simulink model "Simulator_Case_7"  (R2024a)
settings: Solver=VariableStepAuto  StartTime=0.0  StopTime=1000  RelTol=1e-3
values from neighbouring files (symbols this model uses):
  Declination_Sigean = 2.116*(pi/180)    (= 0.0369311669722)    [Parametrization_Simulation_Case_7.m]
  Position_Initial_X = Waypoints_X(1)    [Parametrization_Simulation_Case_7.m]
  Position_Initial_Y = Waypoints_Y(1)    [Parametrization_Simulation_Case_7.m]
  Time_Guidance_Sampling = 20    [Parametrization_Simulation_Case_7.m]
  Time_Period_Sampling = 0.1    [Parametrization_Simulation_Case_7.m]
undefined symbols (not defined in the file or in its folder): Area_Lateral_Projected_Wind, Damping_Factor_Waves, Density_Air, Gain_Derivative, Gain_Filter, Gain_Proportional, Inertia_Moment, Length_Ship, Pulsation_Wave, Rudder_Angle_Maximal, Rudder_Angle_Minimal, Rudder_Rate_Maximal, Rudder_Rate_Minimal, Static_Gain_Nomoto, Structure_Wind_Coefficient, Time_Constant_Total, Velocity_Ship_Mean, Wave_Transfer_Function_Discrete, Waypoints, Yaw_Control_Hydrodynamics_Derivative
libraries: simulink_extras x6, cstblocks x2, sensorgpslib x1, sensorinslib x1
(part 1 of 2)
settings Model: Creator=gerar  LastModifiedBy=gerar

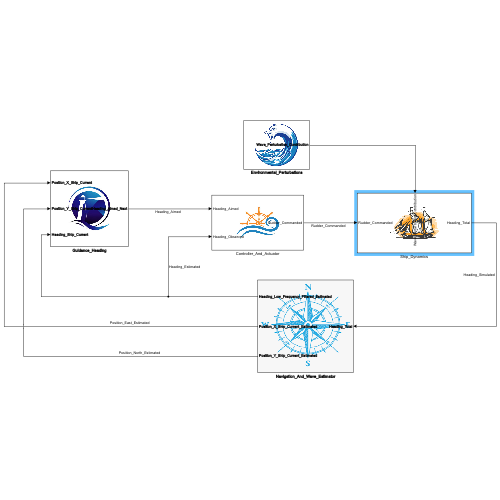
[thumbnail: Simulink's stored preview of the top-level diagram]
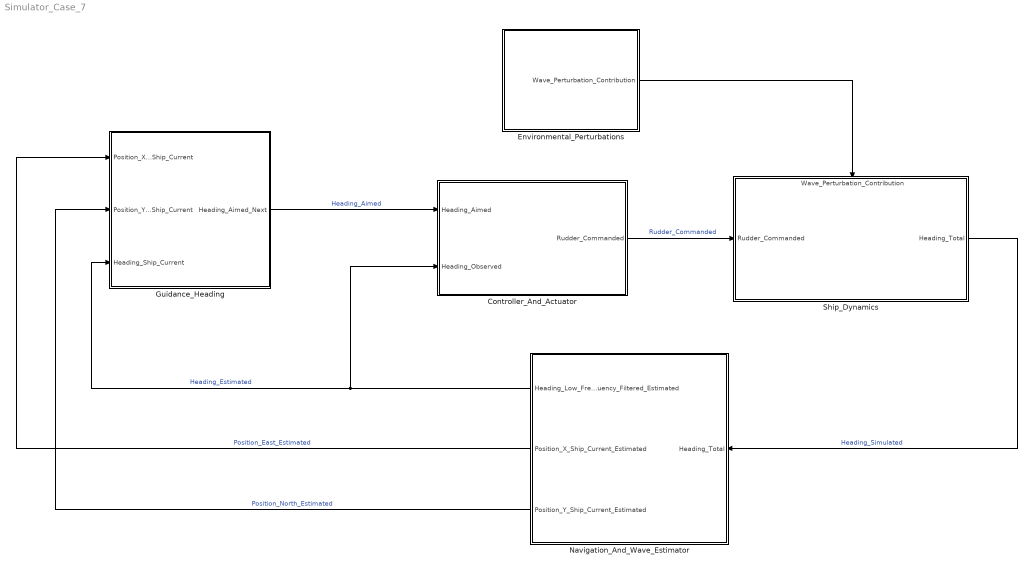
== system Simulator_Case_7 ==
  Controller_And_Actuator : Subsystem
      mask Display: image('Rudder3.jpg');
  Environmental_Perturbations : Subsystem
      mask Display: image('Wave2.png');
  Guidance_Heading : Subsystem
      mask Display: image('phare4.jpg');
  Navigation_And_Wave_Estimator : Subsystem
      mask Display: image('compass4.png');
  Ship_Dynamics : Subsystem
      settings: PortSchema="{\"entries\":[{\"content\":{\"sides\":[{\"content\":{\"connectorIds\":[\"In1\"]},\"type\":\"ConnectorPlacement.EquallySpacedRectSide\",\"uuid\":\"1262d93f-9737-49c5-b1c8-13d3f825160d\"},{\"content\":{\"connectorIds\":[\"Out1\"],\"side\":\"RIGHT\"},\"type\":\"ConnectorPlacement.EquallySpacedRectSide\",\"uuid\":\"2783823e-17f0-4da0-9b4a-e84aa912eb5f\"},{\"content\":{\"connectorIds\":[\"In2\"],\"side\":\"TOP\"},\"type\":\"ConnectorPlacement.EquallySpacedRectSide\",\"uuid\":\"9227960a-c500-4bd1-9392-f2e1de824969\"}]},\"type\":\"ConnectorPlacement.EquallySpacedConnector\",\"uuid\":\"fe1a7a14-057d-49da-982c-994c0d128614\"}],\"packageUris\":[\"http://schema.mathworks.com/mf0/Connector/R2020b\"],\"version\":\"1.0\"}"
      mask Display: image('ship2.png');
  wires:
  Guidance_Heading/1(Heading_Aimed_Next) -> Controller_And_Actuator/1(Heading_Aimed)  "Heading_Aimed"
  Navigation_And_Wave_Estimator/1(Heading_Low_Frequency_Filtered_Estimated) -> Controller_And_Actuator/2(Heading_Observed), Guidance_Heading/3(Heading_Ship_Current)  "Heading_Estimated"
  Environmental_Perturbations/1(Wave_Perturbation_Contribution) -> Ship_Dynamics/2(Wave_Perturbation_Contribution)
  Ship_Dynamics/1(Heading_Total) -> Navigation_And_Wave_Estimator/1(Heading_Total)  "Heading_Simulated"
  Navigation_And_Wave_Estimator/3(Position_Y_Ship_Current_Estimated) -> Guidance_Heading/2(Position_Y_Ship_Current)  "Position_North_Estimated"
  Navigation_And_Wave_Estimator/2(Position_X_Ship_Current_Estimated) -> Guidance_Heading/1(Position_X_Ship_Current)  "Position_East_Estimated"
  Controller_And_Actuator/1(Rudder_Commanded) -> Ship_Dynamics/1(Rudder_Commanded)  "Rudder_Commanded"

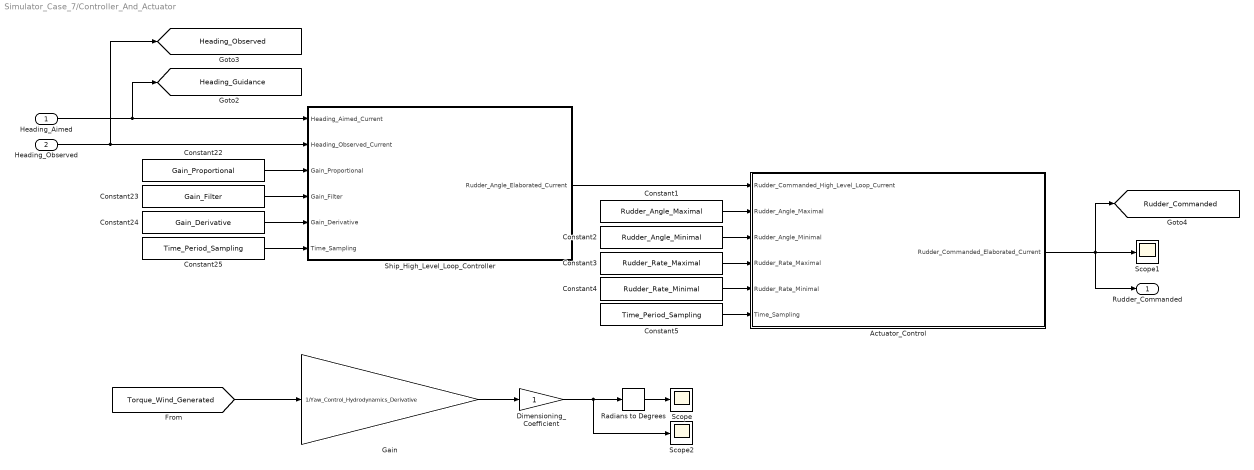
== system Simulator_Case_7/Controller_And_Actuator ==
  Heading_Aimed : Inport
  Heading_Observed : Inport  Port=2
  Actuator_Control : MATLAB Function  TreatAsAtomicUnit=on  SystemSampleTime=Time_Period_Sampling
  Constant1 : Constant  Value=Rudder_Angle_Maximal
  Constant2 : Constant  Value=Rudder_Angle_Minimal
  Constant22 : Constant  Value=Gain_Proportional
  Constant23 : Constant  Value=Gain_Filter
  Constant24 : Constant  Value=Gain_Derivative
  Constant25 : Constant  Value=Time_Period_Sampling
  Constant3 : Constant  Value=Rudder_Rate_Maximal
  Constant4 : Constant  Value=Rudder_Rate_Minimal
  Constant5 : Constant  Value=Time_Period_Sampling
  Dimensioning_Coefficient : Gain
  Gain : Gain  Gain=1/Yaw_Control_Hydrodynamics_Derivative
  Radians to Degrees : simulink_extras/Transformations/Radians to Degrees
  Scope : Scope
  Scope1 : Scope
  Scope2 : Scope
  Ship_High_Level_Loop_Controller : MATLAB Function  TreatAsAtomicUnit=on  SystemSampleTime=Time_Period_Sampling
  Rudder_Commanded : Outport
  tag scope: Heading_Guidance=global, Heading_Observed=global, Rudder_Commanded=global
  wires:
  [Torque_Wind_Generated] -> Gain/1
  Gain/1 -> Dimensioning_Coefficient/1
  Radians to Degrees/1 -> Scope/1
  Dimensioning_Coefficient/1 -> Scope2/1, Radians to Degrees/1
  Heading_Aimed/1 -> Ship_High_Level_Loop_Controller/1(Heading_Aimed_Current), [Heading_Guidance]
  Heading_Observed/1 -> Ship_High_Level_Loop_Controller/2(Heading_Observed_Current), [Heading_Observed]
  Constant22/1 -> Ship_High_Level_Loop_Controller/3(Gain_Proportional)
  Constant23/1 -> Ship_High_Level_Loop_Controller/4(Gain_Filter)
  Constant24/1 -> Ship_High_Level_Loop_Controller/5(Gain_Derivative)
  Constant25/1 -> Ship_High_Level_Loop_Controller/6(Time_Sampling)
  Ship_High_Level_Loop_Controller/1(Rudder_Angle_Elaborated_Current) -> Actuator_Control/1(Rudder_Commanded_High_Level_Loop_Current)
  Constant1/1 -> Actuator_Control/2(Rudder_Angle_Maximal)
  Constant2/1 -> Actuator_Control/3(Rudder_Angle_Minimal)
  Constant3/1 -> Actuator_Control/4(Rudder_Rate_Maximal)
  Constant4/1 -> Actuator_Control/5(Rudder_Rate_Minimal)
  Constant5/1 -> Actuator_Control/6(Time_Sampling)
  Actuator_Control/1(Rudder_Commanded_Elaborated_Current) -> Rudder_Commanded/1, [Rudder_Commanded], Scope1/1

== system Simulator_Case_7/Environmental_Perturbations ==
  Gain : Gain
  Gain1 : Gain
  Wave-Induced_Perturbation_Motion : Subsystem
  Wind_Perturbation_Torque : Subsystem
  Wave_Perturbation_Contribution : Outport
  tag scope: Torque_Wind_Generated=global
  wires:
  Wave-Induced_Perturbation_Motion/1(Wave_Induced_Heading) -> Gain/1
  Gain/1 -> Wave_Perturbation_Contribution/1
  Wind_Perturbation_Torque/1(Torque_Wind) -> Gain1/1
  Gain1/1 -> [Torque_Wind_Generated]

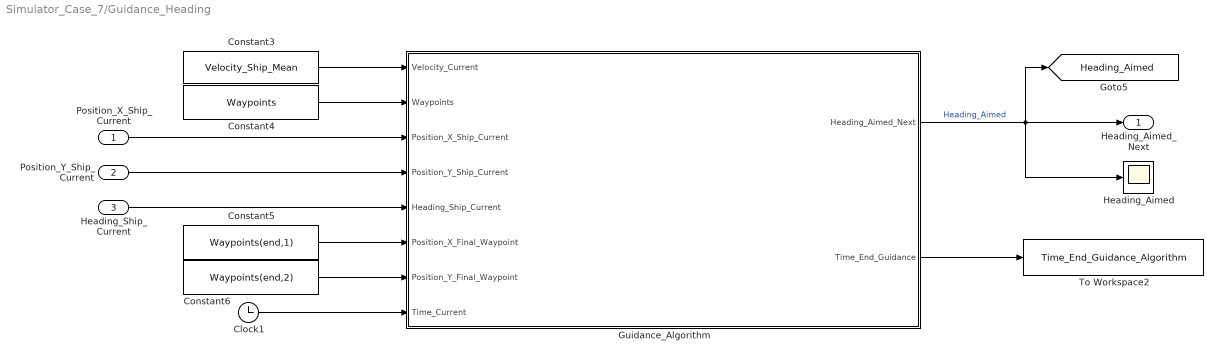
== system Simulator_Case_7/Guidance_Heading ==
  Position_X_Ship_Current : Inport
  Position_Y_Ship_Current : Inport  Port=2
  Heading_Ship_Current : Inport  Port=3
  Clock1 : Clock
  Constant3 : Constant  Value=Velocity_Ship_Mean
  Constant4 : Constant  Value=Waypoints
  Constant5 : Constant  Value=Waypoints(end,1)
  Constant6 : Constant  Value=Waypoints(end,2)
  Guidance_Algorithm : MATLAB Function  TreatAsAtomicUnit=on  SystemSampleTime=Time_Guidance_Sampling*3
  Heading_Aimed : Scope
  To Workspace2 : ToWorkspace  VariableName=Time_End_Guidance_Algorithm  SaveFormat=Timeseries  SampleTime=-1
  Heading_Aimed_Next : Outport
  tag scope: Heading_Aimed=global
  wires:
  Constant5/1 -> Guidance_Algorithm/6(Position_X_Final_Waypoint)
  Guidance_Algorithm/2(Time_End_Guidance) -> To Workspace2/1
  Constant3/1 -> Guidance_Algorithm/1(Velocity_Current)
  Position_Y_Ship_Current/1 -> Guidance_Algorithm/4(Position_Y_Ship_Current)
  Constant4/1 -> Guidance_Algorithm/2(Waypoints)
  Clock1/1 -> Guidance_Algorithm/8(Time_Current)
  Constant6/1 -> Guidance_Algorithm/7(Position_Y_Final_Waypoint)
  Position_X_Ship_Current/1 -> Guidance_Algorithm/3(Position_X_Ship_Current)
  Heading_Ship_Current/1 -> Guidance_Algorithm/5(Heading_Ship_Current)
  Guidance_Algorithm/1(Heading_Aimed_Next) -> Heading_Aimed/1, Heading_Aimed_Next/1, [Heading_Aimed]  "Heading_Aimed"

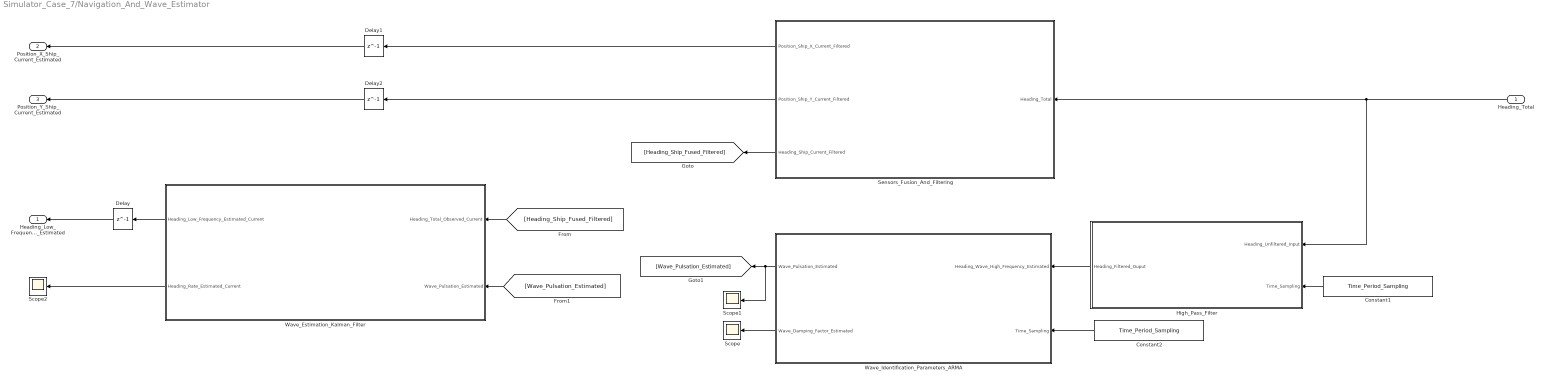
== system Simulator_Case_7/Navigation_And_Wave_Estimator ==
  Heading_Total : Inport
  Constant1 : Constant  Value=Time_Period_Sampling
  Constant2 : Constant  Value=Time_Period_Sampling
  Delay : Delay  DelayLength=1  InputProcessing=Columns as channels (frame based)  SampleTime=Time_Period_Sampling
  Delay1 : Delay  DelayLength=1  InputProcessing=Columns as channels (frame based)  SampleTime=Time_Period_Sampling
  Delay2 : Delay  DelayLength=1  InputProcessing=Columns as channels (frame based)  SampleTime=Time_Period_Sampling
  High_Pass_Filter : MATLAB Function  TreatAsAtomicUnit=on  SystemSampleTime=Time_Period_Sampling
  Scope : Scope
  Scope1 : Scope
  Scope2 : Scope
  Sensors_Fusion_And_Filtering : Subsystem
  Wave_Estimation_Kalman_Filter : Subsystem
  Wave_Identification_Parameters_ARMA : MATLAB Function  TreatAsAtomicUnit=on  SystemSampleTime=Time_Period_Sampling
  Heading_Low_Frequency_Filtered_Estimated : Outport
  Position_X_Ship_Current_Estimated : Outport  Port=2
  Position_Y_Ship_Current_Estimated : Outport  Port=3
  wires:
  Delay1/1 -> Position_X_Ship_Current_Estimated/1
  Delay2/1 -> Position_Y_Ship_Current_Estimated/1
  Sensors_Fusion_And_Filtering/1(Position_Ship_X_Current_Filtered) -> Delay1/1
  Sensors_Fusion_And_Filtering/2(Position_Ship_Y_Current_Filtered) -> Delay2/1
  Wave_Estimation_Kalman_Filter/1(Heading_Low_Frequency_Estimated_Current) -> Delay/1
  High_Pass_Filter/1(Heading_Filtered_Ouput) -> Wave_Identification_Parameters_ARMA/1(Heading_Wave_High_Frequency_Estimated)
  Constant1/1 -> High_Pass_Filter/2(Time_Sampling)
  Heading_Total/1 -> High_Pass_Filter/1(Heading_Unfiltered_Input), Sensors_Fusion_And_Filtering/1(Heading_Total)
  Delay/1 -> Heading_Low_Frequency_Filtered_Estimated/1
  Wave_Estimation_Kalman_Filter/2(Heading_Rate_Estimated_Current) -> Scope2/1
  Constant2/1 -> Wave_Identification_Parameters_ARMA/2(Time_Sampling)
  Sensors_Fusion_And_Filtering/3(Heading_Ship_Current_Filtered) -> [Heading_Ship_Fused_Filtered]
  [Heading_Ship_Fused_Filtered] -> Wave_Estimation_Kalman_Filter/1(Heading_Total_Observed_Current)
  Wave_Identification_Parameters_ARMA/1(Wave_Pulsation_Estimated) -> Scope1/1, [Wave_Pulsation_Estimated]
  [Wave_Pulsation_Estimated] -> Wave_Estimation_Kalman_Filter/2(Wave_Pulsation_Estimated)
  Wave_Identification_Parameters_ARMA/2(Wave_Damping_Factor_Estimated) -> Scope/1

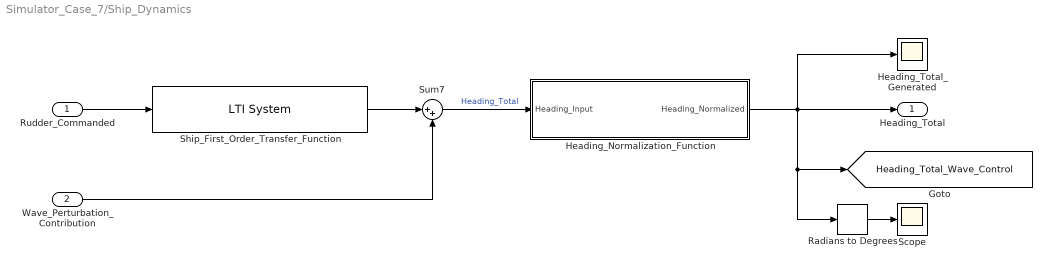
== system Simulator_Case_7/Ship_Dynamics ==
  Rudder_Commanded : Inport
  Wave_Perturbation_Contribution : Inport  Port=2
  Heading_Normalization_Function : MATLAB Function  TreatAsAtomicUnit=on
  Heading_Total_Generated : Scope
  Radians to Degrees : simulink_extras/Transformations/Radians to Degrees
  Scope : Scope
  Ship_First_Order_Transfer_Function : cstblocks/LTI System  sys=Heading_On_Rudder_Transfer_First_Order  IC=[]  PadeOrder=0
  Sum7 : Sum  Inputs=|++
  Heading_Total : Outport
  tag scope: Heading_Total_Wave_Control=global
  wires:
  Wave_Perturbation_Contribution/1 -> Sum7/2
  Rudder_Commanded/1 -> Ship_First_Order_Transfer_Function/1
  Sum7/1 -> Heading_Normalization_Function/1(Heading_Input)  "Heading_Total"
  Radians to Degrees/1 -> Scope/1
  Heading_Normalization_Function/1(Heading_Normalized) -> Radians to Degrees/1, [Heading_Total_Wave_Control], Heading_Total_Generated/1, Heading_Total/1
  Ship_First_Order_Transfer_Function/1 -> Sum7/1

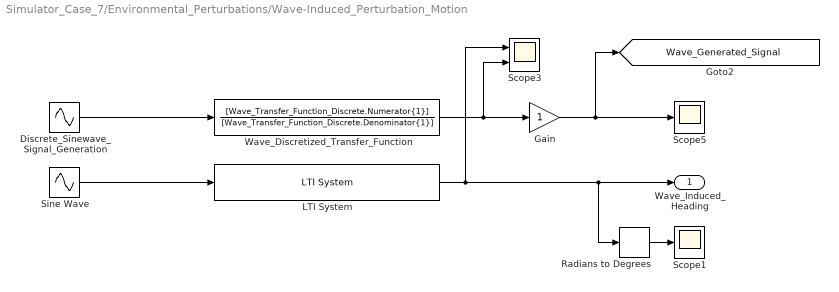
== system Simulator_Case_7/Environmental_Perturbations/Wave-Induced_Perturbation_Motion ==
  Discrete_Sinewave_Signal_Generation : Sin  Amplitude=2*(pi/180)  Frequency=Pulsation_Wave  SampleTime=Time_Period_Sampling
  Gain : Gain
  LTI System : cstblocks/LTI System  sys=Wave_Transfer_Function  IC=[]  PadeOrder=0
  Radians to Degrees : simulink_extras/Transformations/Radians to Degrees
  Scope1 : Scope
  Scope3 : Scope  NumInputPorts=2
  Scope5 : Scope
  Sine Wave : Sin  Amplitude=2*(pi/180)  Frequency=Pulsation_Wave  SampleTime=0
  Wave_Discretized_Transfer_Function : DiscreteTransferFcn  Numerator=[Wave_Transfer_Function_Discrete.Numerator{1}]  Denominator=[Wave_Transfer_Function_Discrete.Denominator{1}]
  Wave_Induced_Heading : Outport
  tag scope: Wave_Generated_Signal=global
  wires:
  Gain/1 -> Scope5/1, [Wave_Generated_Signal]
  Discrete_Sinewave_Signal_Generation/1 -> Wave_Discretized_Transfer_Function/1
  Wave_Discretized_Transfer_Function/1 -> Scope3/2, Gain/1
  Radians to Degrees/1 -> Scope1/1
  Sine Wave/1 -> LTI System/1
  LTI System/1 -> Radians to Degrees/1, Wave_Induced_Heading/1, Scope3/1

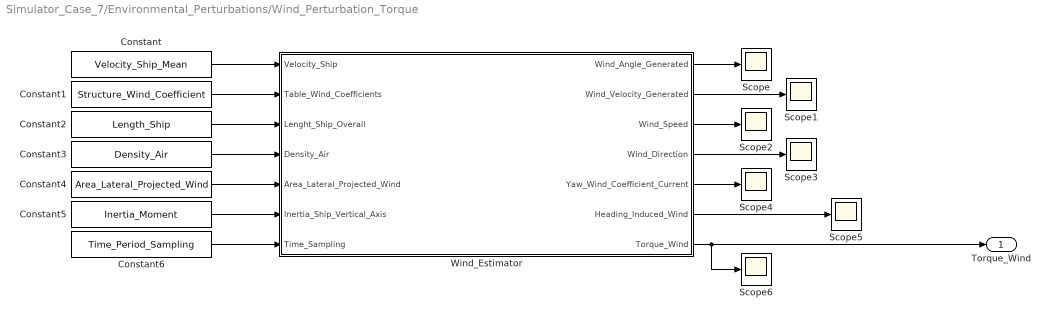
== system Simulator_Case_7/Environmental_Perturbations/Wind_Perturbation_Torque ==
  Constant : Constant  Value=Velocity_Ship_Mean
  Constant1 : Constant  Value=Structure_Wind_Coefficient
  Constant2 : Constant  Value=Length_Ship
  Constant3 : Constant  Value=Density_Air
  Constant4 : Constant  Value=Area_Lateral_Projected_Wind
  Constant5 : Constant  Value=Inertia_Moment
  Constant6 : Constant  Value=Time_Period_Sampling
  Scope{,1..6} (7 alike) : Scope
  Wind_Estimator : MATLAB Function  TreatAsAtomicUnit=on  SystemSampleTime=Time_Period_Sampling
  Torque_Wind : Outport
  wires:
  Wind_Estimator/5(Yaw_Wind_Coefficient_Current) -> Scope4/1
  Constant2/1 -> Wind_Estimator/3(Lenght_Ship_Overall)
  Constant/1 -> Wind_Estimator/1(Velocity_Ship)
  Constant5/1 -> Wind_Estimator/6(Inertia_Ship_Vertical_Axis)
  Constant4/1 -> Wind_Estimator/5(Area_Lateral_Projected_Wind)
  Constant3/1 -> Wind_Estimator/4(Density_Air)
  Wind_Estimator/1(Wind_Angle_Generated) -> Scope/1
  Wind_Estimator/2(Wind_Velocity_Generated) -> Scope1/1
  Wind_Estimator/3(Wind_Speed) -> Scope2/1
  Wind_Estimator/7(Torque_Wind) -> Torque_Wind/1, Scope6/1
  Constant1/1 -> Wind_Estimator/2(Table_Wind_Coefficients)
  Constant6/1 -> Wind_Estimator/7(Time_Sampling)
  Wind_Estimator/6(Heading_Induced_Wind) -> Scope5/1
  Wind_Estimator/4(Wind_Direction) -> Scope3/1

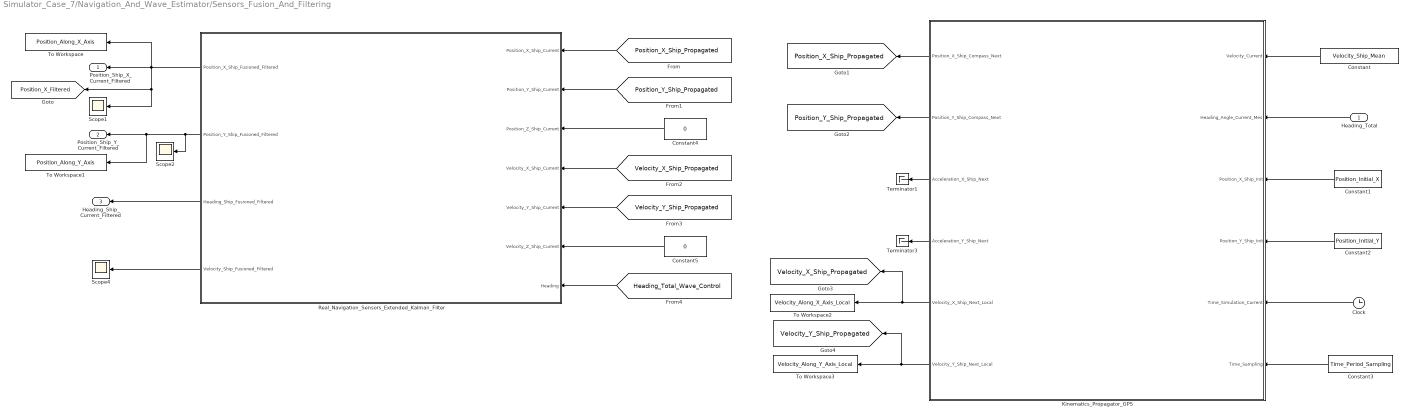
== system Simulator_Case_7/Navigation_And_Wave_Estimator/Sensors_Fusion_And_Filtering ==
  Heading_Total : Inport
  Clock : Clock
  Constant : Constant  Value=Velocity_Ship_Mean
  Constant1 : Constant  Value=Position_Initial_X
  Constant2 : Constant  Value=Position_Initial_Y
  Constant3 : Constant  Value=Time_Period_Sampling
  Constant4 : Constant  Value=0
  Constant5 : Constant  Value=0
  Kinematics_Propagator_GPS : MATLAB Function  TreatAsAtomicUnit=on  SystemSampleTime=Time_Period_Sampling
  Real_Navigation_Sensors_Extended_Kalman_Filter : Subsystem
  Scope1 : Scope
  Scope2 : Scope
  Scope4 : Scope
  Terminator1 : Terminator
  Terminator3 : Terminator
  To Workspace : ToWorkspace  VariableName=Position_Along_X_Axis  SaveFormat=Timeseries  SampleTime=Time_Period_Sampling
  To Workspace1 : ToWorkspace  VariableName=Position_Along_Y_Axis  SaveFormat=Timeseries  SampleTime=Time_Period_Sampling
  To Workspace2 : ToWorkspace  VariableName=Velocity_Along_X_Axis_Local  SaveFormat=Timeseries  SampleTime=Time_Period_Sampling
  To Workspace3 : ToWorkspace  VariableName=Velocity_Along_Y_Axis_Local  SaveFormat=Timeseries  SampleTime=Time_Period_Sampling
  Position_Ship_X_Current_Filtered : Outport
  Position_Ship_Y_Current_Filtered : Outport  Port=2
  Heading_Ship_Current_Filtered : Outport  Port=3
  tag scope: Position_X_Filtered=global, Position_X_Ship_Propagated=global, Position_Y_Ship_Propagated=global, Velocity_X_Ship_Propagated=global, Velocity_Y_Ship_Propagated=global
  wires:
  Constant2/1 -> Kinematics_Propagator_GPS/4(Position_Y_Ship_Init)
  Clock/1 -> Kinematics_Propagator_GPS/5(Time_Simulation_Current)
  Constant1/1 -> Kinematics_Propagator_GPS/3(Position_X_Ship_Init)
  Constant/1 -> Kinematics_Propagator_GPS/1(Velocity_Current)
  Constant3/1 -> Kinematics_Propagator_GPS/6(Time_Sampling)
  Kinematics_Propagator_GPS/3(Acceleration_X_Ship_Next) -> Terminator1/1
  Kinematics_Propagator_GPS/4(Acceleration_Y_Ship_Next) -> Terminator3/1
  Heading_Total/1 -> Kinematics_Propagator_GPS/2(Heading_Angle_Current_Mes)
  Kinematics_Propagator_GPS/5(Velocity_X_Ship_Next_Local) -> [Velocity_X_Ship_Propagated], To Workspace2/1
  Kinematics_Propagator_GPS/6(Velocity_Y_Ship_Next_Local) -> [Velocity_Y_Ship_Propagated], To Workspace3/1
  Kinematics_Propagator_GPS/1(Position_X_Ship_Compass_Next) -> [Position_X_Ship_Propagated]
  Kinematics_Propagator_GPS/2(Position_Y_Ship_Compass_Next) -> [Position_Y_Ship_Propagated]
  [Position_X_Ship_Propagated] -> Real_Navigation_Sensors_Extended_Kalman_Filter/1(Position_X_Ship_Current)
  [Position_Y_Ship_Propagated] -> Real_Navigation_Sensors_Extended_Kalman_Filter/2(Position_Y_Ship_Current)
  Constant4/1 -> Real_Navigation_Sensors_Extended_Kalman_Filter/3(Position_Z_Ship_Current)
  [Velocity_X_Ship_Propagated] -> Real_Navigation_Sensors_Extended_Kalman_Filter/4(Velocity_X_Ship_Current)
  [Velocity_Y_Ship_Propagated] -> Real_Navigation_Sensors_Extended_Kalman_Filter/5(Velocity_Y_Ship_Current)
  Constant5/1 -> Real_Navigation_Sensors_Extended_Kalman_Filter/6(Velocity_Z_Ship_Current)
  [Heading_Total_Wave_Control] -> Real_Navigation_Sensors_Extended_Kalman_Filter/7(Heading)
  Real_Navigation_Sensors_Extended_Kalman_Filter/1(Position_X_Ship_Fusioned_Filtered) -> Position_Ship_X_Current_Filtered/1, To Workspace/1, [Position_X_Filtered], Scope1/1
  Real_Navigation_Sensors_Extended_Kalman_Filter/2(Position_Y_Ship_Fusioned_Filtered) -> Scope2/1, To Workspace1/1, Position_Ship_Y_Current_Filtered/1
  Real_Navigation_Sensors_Extended_Kalman_Filter/3(Heading_Ship_Fusioned_Filtered) -> Heading_Ship_Current_Filtered/1
  Real_Navigation_Sensors_Extended_Kalman_Filter/4(Velocity_Ship_Fusioned_Filtered) -> Scope4/1

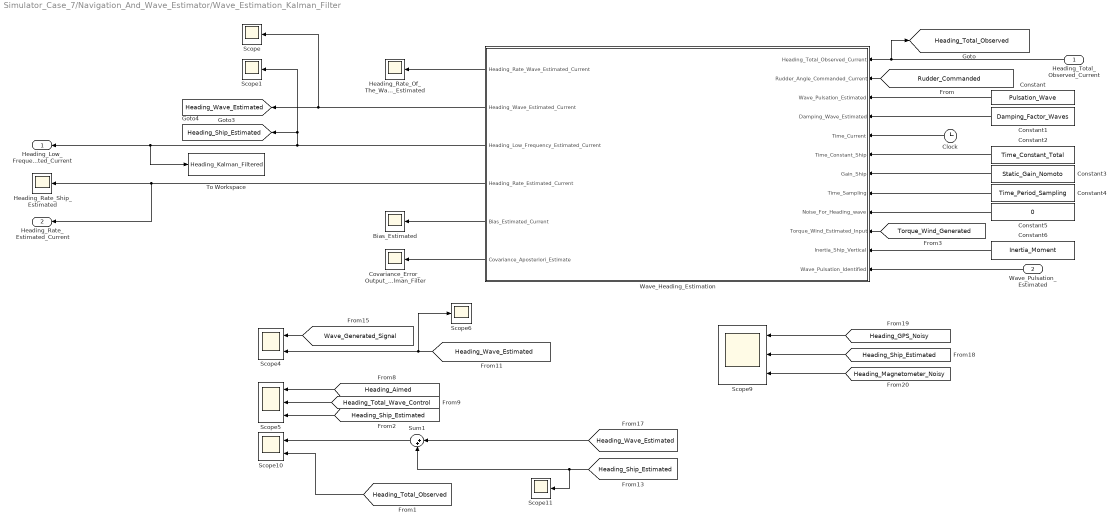
== system Simulator_Case_7/Navigation_And_Wave_Estimator/Wave_Estimation_Kalman_Filter ==
  Heading_Total_Observed_Current : Inport
  Wave_Pulsation_Estimated : Inport  Port=2
  Bias_Estimated : Scope
  Clock : Clock
  Constant : Constant  Value=Pulsation_Wave  SampleTime=Time_Period_Sampling
  Constant1 : Constant  Value=Damping_Factor_Waves  SampleTime=Time_Period_Sampling
  Constant2 : Constant  Value=Time_Constant_Total  SampleTime=Time_Period_Sampling
  Constant3 : Constant  Value=Static_Gain_Nomoto  SampleTime=Time_Period_Sampling
  Constant4 : Constant  Value=Time_Period_Sampling  SampleTime=Time_Period_Sampling
  Constant5 : Constant  Value=0
  Constant6 : Constant  Value=Inertia_Moment
  Covariance_Error_Output_Kalman_Filter : Scope
  Heading_Rate_Of_The_Waves_Estimated : Scope
  Heading_Rate_Ship_Estimated : Scope
  Scope{,1,6,11} (4 alike) : Scope
  Scope10 : Scope  NumInputPorts=2
  Scope4 : Scope  NumInputPorts=2
  Scope5 : Scope  NumInputPorts=3
  Scope9 : Scope  NumInputPorts=3
  Sum1 : Sum  Inputs=|++
  To Workspace : ToWorkspace  VariableName=Heading_Kalman_Filtered  SaveFormat=Timeseries  SampleTime=Time_Period_Sampling
  Wave_Heading_Estimation : MATLAB Function  TreatAsAtomicUnit=on  SystemSampleTime=Time_Period_Sampling
  Heading_Low_Frequency_Estimated_Current : Outport
  Heading_Rate_Estimated_Current : Outport  Port=2
  tag scope: Heading_Ship_Estimated=global, Heading_Total_Observed=global, Heading_Wave_Estimated=global
  wires:
  Wave_Heading_Estimation/3(Heading_Low_Frequency_Estimated_Current) -> Scope1/1, [Heading_Ship_Estimated], Heading_Low_Frequency_Estimated_Current/1, To Workspace/1
  Heading_Total_Observed_Current/1 -> [Heading_Total_Observed], Wave_Heading_Estimation/1(Heading_Total_Observed_Current)
  [Rudder_Commanded] -> Wave_Heading_Estimation/2(Rudder_Angle_Commanded_Current)
  Constant/1 -> Wave_Heading_Estimation/3(Wave_Pulsation_Estimated)
  Constant1/1 -> Wave_Heading_Estimation/4(Damping_Wave_Estimated)
  Clock/1 -> Wave_Heading_Estimation/5(Time_Current)
  Constant2/1 -> Wave_Heading_Estimation/6(Time_Constant_Ship)
  Constant3/1 -> Wave_Heading_Estimation/7(Gain_Ship)
  Constant4/1 -> Wave_Heading_Estimation/8(Time_Sampling)
  Constant5/1 -> Wave_Heading_Estimation/9(Noise_For_Heading_wave)
  Wave_Heading_Estimation/1(Heading_Rate_Wave_Estimated_Current) -> Heading_Rate_Of_The_Waves_Estimated/1
  Wave_Heading_Estimation/2(Heading_Wave_Estimated_Current) -> Scope/1, [Heading_Wave_Estimated]
  Wave_Heading_Estimation/5(Bias_Estimated_Current) -> Bias_Estimated/1
  Wave_Heading_Estimation/4(Heading_Rate_Estimated_Current) -> Heading_Rate_Estimated_Current/1, Heading_Rate_Ship_Estimated/1
  Wave_Heading_Estimation/6(Covariance_Aposteriori_Estimate) -> Covariance_Error_Output_Kalman_Filter/1
  [Heading_Aimed] -> Scope5/1
  [Wave_Generated_Signal] -> Scope4/1
  [Heading_Ship_Estimated] -> Scope9/2
  [Heading_Magnetometer_Noisy] -> Scope9/3
  [Heading_Ship_Estimated] -> Scope11/1, Sum1/2
  [Heading_GPS_Noisy] -> Scope9/1
  [Heading_Wave_Estimated] -> Sum1/1
  Sum1/1 -> Scope10/1
  [Heading_Total_Wave_Control] -> Scope5/2
  [Heading_Ship_Estimated] -> Scope5/3
  [Heading_Wave_Estimated] -> Scope6/1, Scope4/2
  [Heading_Total_Observed] -> Scope10/2
  Constant6/1 -> Wave_Heading_Estimation/11(Inertia_Ship_Vertical)
  [Torque_Wind_Generated] -> Wave_Heading_Estimation/10(Torque_Wind_Estimated_Input)
  Wave_Pulsation_Estimated/1 -> Wave_Heading_Estimation/12(Wave_Pulsation_Identified)

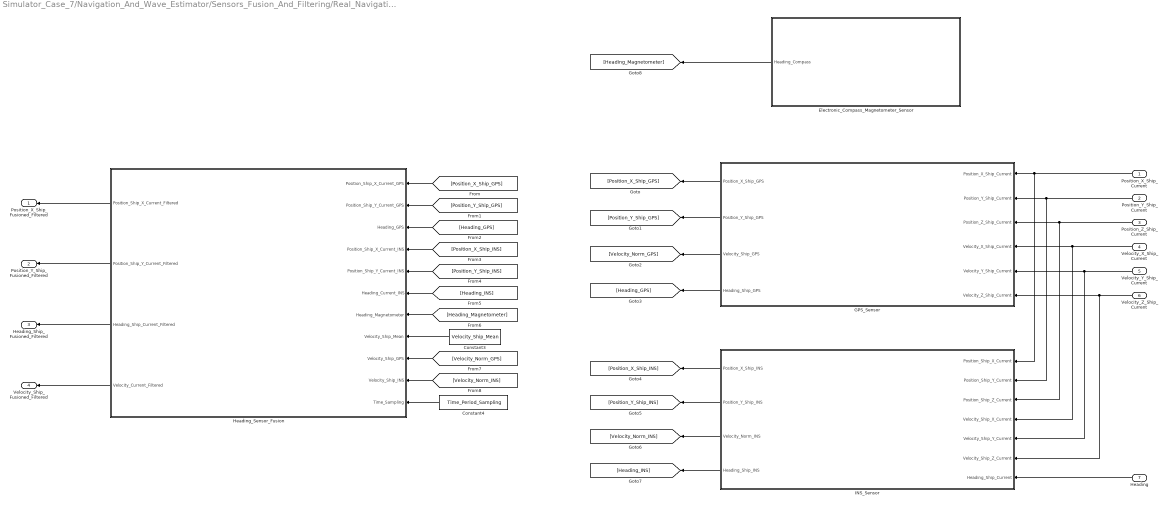
== system Simulator_Case_7/Navigation_And_Wave_Estimator/Sensors_Fusion_And_Filtering/Real_Navigation_Sensors_Extended_Kalman_Filter ==
  Position_X_Ship_Current : Inport
  Position_Y_Ship_Current : Inport  Port=2
  Position_Z_Ship_Current : Inport  Port=3
  Velocity_X_Ship_Current : Inport  Port=4
  Velocity_Y_Ship_Current : Inport  Port=5
  Velocity_Z_Ship_Current : Inport  Port=6
  Heading : Inport  Port=7
  Constant3 : Constant  Value=Velocity_Ship_Mean
  Constant4 : Constant  Value=Time_Period_Sampling
  Electronic_Compass_Magnetometer_Sensor : Subsystem
  GPS_Sensor : Subsystem
  Heading_Sensor_Fusion : MATLAB Function  TreatAsAtomicUnit=on  SystemSampleTime=Time_Period_Sampling
  INS_Sensor : Subsystem
  Position_X_Ship_Fusioned_Filtered : Outport
  Position_Y_Ship_Fusioned_Filtered : Outport  Port=2
  Heading_Ship_Fusioned_Filtered : Outport  Port=3
  Velocity_Ship_Fusioned_Filtered : Outport  Port=4
  wires:
  Electronic_Compass_Magnetometer_Sensor/1(Heading_Compass) -> [Heading_Magnetometer]
  Position_Z_Ship_Current/1 -> INS_Sensor/3(Position_Ship_Z_Current), GPS_Sensor/3(Position_Z_Ship_Current)
  Velocity_Z_Ship_Current/1 -> INS_Sensor/6(Velocity_Ship_Z_Current), GPS_Sensor/6(Velocity_Z_Ship_Current)
  GPS_Sensor/1(Position_X_Ship_GPS) -> [Position_X_Ship_GPS]
  GPS_Sensor/2(Position_Y_Ship_GPS) -> [Position_Y_Ship_GPS]
  GPS_Sensor/3(Velocity_Ship_GPS) -> [Velocity_Norm_GPS]
  GPS_Sensor/4(Heading_Ship_GPS) -> [Heading_GPS]
  Position_X_Ship_Current/1 -> INS_Sensor/1(Position_Ship_X_Current), GPS_Sensor/1(Position_X_Ship_Current)
  Velocity_X_Ship_Current/1 -> INS_Sensor/4(Velocity_Ship_X_Current), GPS_Sensor/4(Velocity_X_Ship_Current)
  Velocity_Y_Ship_Current/1 -> INS_Sensor/5(Velocity_Ship_Y_Current), GPS_Sensor/5(Velocity_Y_Ship_Current)
  Position_Y_Ship_Current/1 -> INS_Sensor/2(Position_Ship_Y_Current), GPS_Sensor/2(Position_Y_Ship_Current)
  Heading/1 -> INS_Sensor/7(Heading_Ship_Current)
  INS_Sensor/1(Position_X_Ship_INS) -> [Position_X_Ship_INS]
  INS_Sensor/2(Position_Y_Ship_INS) -> [Position_Y_Ship_INS]
  INS_Sensor/3(Velocity_Norm_INS) -> [Velocity_Norm_INS]
  INS_Sensor/4(Heading_Ship_INS) -> [Heading_INS]
  Constant3/1 -> Heading_Sensor_Fusion/8(Velocity_Ship_Mean)
  Constant4/1 -> Heading_Sensor_Fusion/11(Time_Sampling)
  [Position_X_Ship_GPS] -> Heading_Sensor_Fusion/1(Position_Ship_X_Current_GPS)
  [Position_Y_Ship_GPS] -> Heading_Sensor_Fusion/2(Position_Ship_Y_Current_GPS)
  [Heading_GPS] -> Heading_Sensor_Fusion/3(Heading_GPS)
  [Position_X_Ship_INS] -> Heading_Sensor_Fusion/4(Position_Ship_X_Current_INS)
  [Position_Y_Ship_INS] -> Heading_Sensor_Fusion/5(Position_Ship_Y_Current_INS)
  [Heading_INS] -> Heading_Sensor_Fusion/6(Heading_Current_INS)
  [Heading_Magnetometer] -> Heading_Sensor_Fusion/7(Heading_Magnetometer)
  [Velocity_Norm_GPS] -> Heading_Sensor_Fusion/9(Velocity_Ship_GPS)
  [Velocity_Norm_INS] -> Heading_Sensor_Fusion/10(Velocity_Ship_INS)
  Heading_Sensor_Fusion/1(Position_Ship_X_Current_Filtered) -> Position_X_Ship_Fusioned_Filtered/1
  Heading_Sensor_Fusion/2(Position_Ship_Y_Current_Filtered) -> Position_Y_Ship_Fusioned_Filtered/1
  Heading_Sensor_Fusion/3(Heading_Ship_Current_Filtered) -> Heading_Ship_Fusioned_Filtered/1
  Heading_Sensor_Fusion/4(Velocity_Current_Filtered) -> Velocity_Ship_Fusioned_Filtered/1

== system Simulator_Case_7/Navigation_And_Wave_Estimator/Sensors_Fusion_And_Filtering/Real_Navigation_Sensors_Extended_Kalman_Filter/Electronic_Compass_Magnetometer_Sensor ==
  Constant : Constant  Value=Declination_Sigean
  Scope8 : Scope
  Sum : Sum  Inputs=|++
  To Workspace1 : ToWorkspace  VariableName=Heading_Noisy_Magnetometer  SaveFormat=Timeseries  SampleTime=Time_Period_Sampling
  Heading_Compass : Outport
  tag scope: Heading_Magnetometer_Noisy=global
  wires:
  Sum/1 -> Heading_Compass/1, Scope8/1, To Workspace1/1, [Heading_Magnetometer_Noisy]
  Constant/1 -> Sum/1
  [Heading_Total_Wave_Control] -> Sum/2

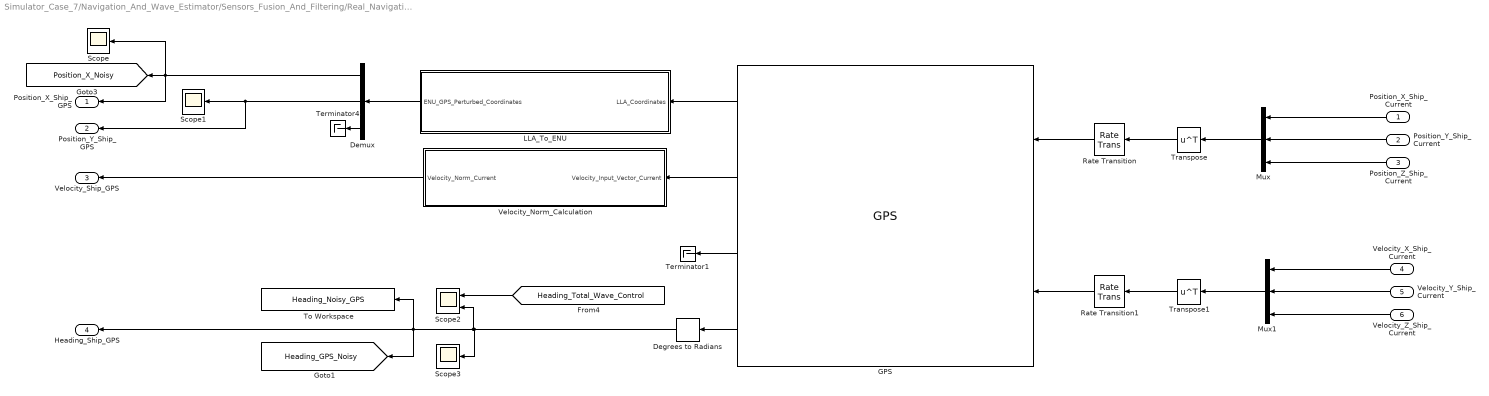
== system Simulator_Case_7/Navigation_And_Wave_Estimator/Sensors_Fusion_And_Filtering/Real_Navigation_Sensors_Extended_Kalman_Filter/GPS_Sensor ==
  Position_X_Ship_Current : Inport
  Position_Y_Ship_Current : Inport  Port=2
  Position_Z_Ship_Current : Inport  Port=3
  Velocity_X_Ship_Current : Inport  Port=4
  Velocity_Y_Ship_Current : Inport  Port=5
  Velocity_Z_Ship_Current : Inport  Port=6
  Degrees to Radians : simulink_extras/Transformations/Degrees to Radians
  Demux : Demux  Outputs=3
  GPS : sensorgpslib/GPS  DispRefFrame=ENU  PositionInputFormat=Local  ReferenceLocation=[43.059023, 3.002915 ,0]  HorizontalPositionAccuracy=2  VerticalPositionAccuracy=2  VelocityAccuracy=0.1  DecayFactor=0.999  SeedDouble=67  SimulateUsing=Interpreted execution
  LLA_To_ENU : MATLAB Function  TreatAsAtomicUnit=on  SystemSampleTime=Time_Period_Sampling
  Mux : Mux  Inputs=3
  Mux1 : Mux  Inputs=3
  Rate Transition : RateTransition  OutPortSampleTime=Time_Period_Sampling
  Rate Transition1 : RateTransition  OutPortSampleTime=Time_Period_Sampling
  Scope : Scope
  Scope1 : Scope
  Scope2 : Scope  NumInputPorts=2
  Scope3 : Scope
  Terminator1 : Terminator
  Terminator4 : Terminator
  To Workspace : ToWorkspace  VariableName=Heading_Noisy_GPS  SaveFormat=Timeseries  SampleTime=Time_Period_Sampling
  Transpose : Math  Operator=transpose
  Transpose1 : Math  Operator=transpose
  Velocity_Norm_Calculation : MATLAB Function  TreatAsAtomicUnit=on
  Position_X_Ship_GPS : Outport
  Position_Y_Ship_GPS : Outport  Port=2
  Velocity_Ship_GPS : Outport  Port=3
  Heading_Ship_GPS : Outport  Port=4
  tag scope: Heading_GPS_Noisy=global, Position_X_Noisy=global
  wires:
  Degrees to Radians/1 -> Heading_Ship_GPS/1, [Heading_GPS_Noisy], To Workspace/1, Scope2/2, Scope3/1
  Demux/1 -> Scope/1, [Position_X_Noisy], Position_X_Ship_GPS/1
  Transpose1/1 -> Rate Transition1/1
  Velocity_Norm_Calculation/1(Velocity_Norm_Current) -> Velocity_Ship_GPS/1
  Demux/2 -> Scope1/1, Position_Y_Ship_GPS/1
  Position_Z_Ship_Current/1 -> Mux/3
  Transpose/1 -> Rate Transition/1
  Position_X_Ship_Current/1 -> Mux/1
  GPS/1 -> LLA_To_ENU/1(LLA_Coordinates)
  Rate Transition1/1 -> GPS/2
  Velocity_X_Ship_Current/1 -> Mux1/1
  Demux/3 -> Terminator4/1
  LLA_To_ENU/1(ENU_GPS_Perturbed_Coordinates) -> Demux/1
  Mux/1 -> Transpose/1
  GPS/3 -> Terminator1/1
  GPS/4 -> Degrees to Radians/1
  Mux1/1 -> Transpose1/1
  [Heading_Total_Wave_Control] -> Scope2/1
  GPS/2 -> Velocity_Norm_Calculation/1(Velocity_Input_Vector_Current)
  Rate Transition/1 -> GPS/1
  Position_Y_Ship_Current/1 -> Mux/2
  Velocity_Y_Ship_Current/1 -> Mux1/2
  Velocity_Z_Ship_Current/1 -> Mux1/3

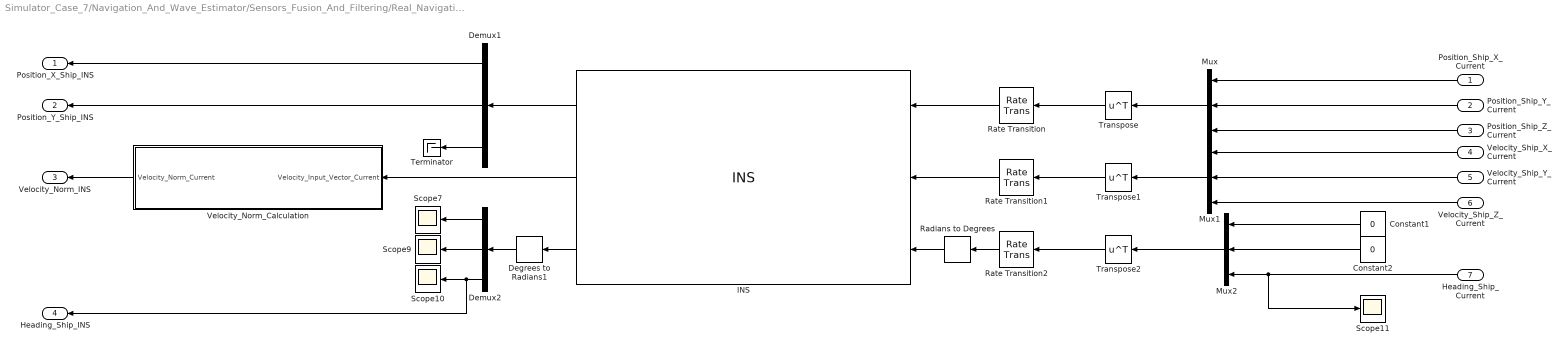
== system Simulator_Case_7/Navigation_And_Wave_Estimator/Sensors_Fusion_And_Filtering/Real_Navigation_Sensors_Extended_Kalman_Filter/INS_Sensor ==
  Position_Ship_X_Current : Inport
  Position_Ship_Y_Current : Inport  Port=2
  Position_Ship_Z_Current : Inport  Port=3
  Velocity_Ship_X_Current : Inport  Port=4
  Velocity_Ship_Y_Current : Inport  Port=5
  Velocity_Ship_Z_Current : Inport  Port=6
  Heading_Ship_Current : Inport  Port=7
  Constant1 : Constant  Value=0
  Constant2 : Constant  Value=0
  Degrees to Radians1 : simulink_extras/Transformations/Degrees to Radians
  Demux1 : Demux  Outputs=3
  Demux2 : Demux  Outputs=3
  INS : sensorinslib/INS  MountingLocation=[0 0 0]  RollAccuracy=0.2  PitchAccuracy=0.2  YawAccuracy=0.5  PositionAccuracy=1  VelocityAccuracy=0.2  UseAccelAndAngVel=off  AccelerationAccuracy=0  AngularVelocityAccuracy=0  TimeInput=off  PositionErrorFactor=[0 0 0]  SeedDouble=67  SimulateUsing=Code generation
      settings: LibrarySourceBlock=mspsensorlib/INS
  Mux : Mux  Inputs=3
  Mux1 : Mux  Inputs=3
  Mux2 : Mux  Inputs=3
  Radians to Degrees : simulink_extras/Transformations/Radians to Degrees
  Rate Transition : RateTransition  OutPortSampleTime=Time_Period_Sampling
  Rate Transition1 : RateTransition  OutPortSampleTime=Time_Period_Sampling
  Rate Transition2 : RateTransition  OutPortSampleTime=Time_Period_Sampling
  Scope{7,9..11} (4 alike) : Scope
  Terminator : Terminator
  Transpose : Math  Operator=transpose
  Transpose1 : Math  Operator=transpose
  Transpose2 : Math  Operator=transpose
  Velocity_Norm_Calculation : MATLAB Function  TreatAsAtomicUnit=on
  Position_X_Ship_INS : Outport
  Position_Y_Ship_INS : Outport  Port=2
  Velocity_Norm_INS : Outport  Port=3
  Heading_Ship_INS : Outport  Port=4
  wires:
  Heading_Ship_Current/1 -> Scope11/1, Mux2/3
  Radians to Degrees/1 -> INS/3
  Position_Ship_X_Current/1 -> Mux/1
  Mux/1 -> Transpose/1
  Transpose/1 -> Rate Transition/1
  Velocity_Ship_Y_Current/1 -> Mux1/2
  Rate Transition2/1 -> Radians to Degrees/1
  Transpose2/1 -> Rate Transition2/1
  Constant1/1 -> Mux2/1
  INS/3 -> Degrees to Radians1/1
  Position_Ship_Y_Current/1 -> Mux/2
  Demux2/3 -> Heading_Ship_INS/1, Scope10/1
  Demux2/1 -> Scope7/1
  INS/2 -> Velocity_Norm_Calculation/1(Velocity_Input_Vector_Current)
  Position_Ship_Z_Current/1 -> Mux/3
  Constant2/1 -> Mux2/2
  Velocity_Ship_X_Current/1 -> Mux1/1
  Demux2/2 -> Scope9/1
  Mux2/1 -> Transpose2/1
  Demux1/2 -> Position_Y_Ship_INS/1
  Degrees to Radians1/1 -> Demux2/1
  Demux1/1 -> Position_X_Ship_INS/1
  Mux1/1 -> Transpose1/1
  INS/1 -> Demux1/1
  Rate Transition/1 -> INS/1
  Transpose1/1 -> Rate Transition1/1
  Rate Transition1/1 -> INS/2
  Velocity_Norm_Calculation/1(Velocity_Norm_Current) -> Velocity_Norm_INS/1
  Velocity_Ship_Z_Current/1 -> Mux1/3
  Demux1/3 -> Terminator/1

== matlab function Simulator_Case_7/Navigation_And_Wave_Estimator/Sensors_Fusion_And_Filtering/Real_Navigation_Sensors_Extended_Kalman_Filter/Heading_Sensor_Fusion ==
  settings: updateMethod=DISCRETE
  data: Position_Ship_X_Current_GPS input; Position_Ship_Y_Current_GPS input; Heading_GPS input; Position_Ship_X_Current_INS input; Position_Ship_Y_Current_INS input; Heading_Current_INS input; Heading_Magnetometer input; Position_Ship_X_Current_Filtered output; Position_Ship_Y_Current_Filtered output; Heading_Ship_Current_Filtered output; Velocity_Current_Filtered output; Velocity_Ship_Mean input; Velocity_Ship_GPS input; Velocity_Ship_INS input; Time_Sampling input
function [Position_Ship_X_Current_Filtered,...
          Position_Ship_Y_Current_Filtered,...
          Heading_Ship_Current_Filtered,...
          Velocity_Current_Filtered] = Navigation_Kalman_Sensor_Fusion(Position_Ship_X_Current_GPS,...
                                                                       Position_Ship_Y_Current_GPS,...
                                                                       Heading_GPS,...
                                                                       Position_Ship_X_Current_INS,...
                                                                       Position_Ship_Y_Current_INS,...
                                                                       Heading_Current_INS,...
                                                                       Heading_Magnetometer,...
                                                                       Velocity_Ship_Mean,...
                                                                       Velocity_Ship_GPS,...
                                                                       Velocity_Ship_INS,...
                                                                       Time_Sampling)

% This function serves as a filtering and data fusion to provide the ship
% with the right heading data.

persistent State_Model_Prediction;
persistent Covariance_Model_Prediction;

% ----------------------------------------------------------------
% 1) Definition of the process model:
% ----------------------------------------------------------------
% Initialization of the current models:
Position_Ship_X_Current_Model = Position_Ship_X_Current_GPS;
Position_Ship_Y_Current_Model = Position_Ship_Y_Current_GPS;
Heading_Current_Model = Heading_Magnetometer;
Velocity_Ship_Model = Velocity_Ship_Mean;
States_Initial_Model = [Position_Ship_X_Current_Model;...
                        Position_Ship_Y_Current_Model;...
                        Heading_Current_Model;...
                        Velocity_Ship_Model];

% We then define the process noise covariance matrix refered as the 'Q'
% matrix in estimation. This has a link with how one is confident about the
% used model:
Variance_Position_X = 5;
Variance_Position_Y = 5;
Variance_Heading = (2*pi/180);
Variance_Velocity = 0.5;
Process_Model_Covariance_Matrix = [Variance_Position_X^2 0 0 0;
                                   0 Variance_Position_Y^2 0 0;
                                   0 0 Variance_Heading^2 0;
                                   0 0 0 Variance_Velocity^2];

% Compute the covariance matrix of the states at the initial step refered as the 'P0|0':
Covariance_States_Initial_Model = Process_Model_Covariance_Matrix;

% Compute the control input matrix refered as the 'B' matrix:
Control_Inputs_Initial = 0; % Process model considered as without input influence.

% Time step for numerical integration:
Time_Step_Integration = Time_Sampling;

% ----------------------------------------------------------------
% 2) Measurement & Innovation model:
% ----------------------------------------------------------------
% Definition of the measurement noise covariance matrix refered as 'R' matrix:
Variance_Position_X_GPS = 2;
Variance_Position_Y_GPS = 2;
Variance_Heading_GNSS = 0.1*(pi/180);
Variance_Position_X_INS = 1;
Variance_Position_Y_INS = 1;
Variance_Heading_INS = 0.1*(pi/180);
Variance_Heading_Magnetic = 2*(pi/180);
Variance_Velocity_GPS = 0.1;
Variance_Velocity_INS = 0.2;
Measurement_Covariance_Matrix = [Variance_Position_X_GPS^2 0 0 0 0 0 0 0 0;
                                 0 Variance_Position_Y_GPS^2 0 0 0 0 0 0 0;
                                 0 0 Variance_Heading_GNSS^2 0 0 0 0 0 0;
                                 0 0 0 Variance_Position_X_INS^2 0 0 0 0 0;
                                 0 0 0 0 Variance_Position_Y_INS^2 0 0 0 0;
                                 0 0 0 0 0 Variance_Heading_INS^2 0 0 0;
                                 0 0 0 0 0 0 Variance_Heading_Magnetic^2 0 0;
                                 0 0 0 0 0 0 0 Variance_Velocity_GPS^2 0;
                                 0 0 0 0 0 0 0 0 Variance_Velocity_INS^2];

% Define the measurement model matrix: (often refered as 'H' or 'Gx'
% matrices):
Measurement_Model_Matrix = [1 0 0 0;
                            0 1 0 0;
                            0 0 1 0;
                            1 0 0 0;
                            0 1 0 0;
                            0 0 1 0;
                            0 0 1 0;
                            0 0 0 1;
                            0 0 0 1];

% ----------------------------------------------------------------
% Extended Kalman Filter loop calculations:
% ----------------------------------------------------------------
% Initialization:
if isempty(State_Model_Prediction)
    State_Model_Prediction = States_Initial_Model;
end
States_Previous = State_Model_Prediction; % The 'X' state vector.
if isempty(Covariance_Model_Prediction)
    Covariance_Model_Prediction = Covariance_States_Initial_Model;
end
Covariance_State_Previous = Covariance_Model_Prediction; % The 'P0|0' equal to 'Q' in this case.
Control_Inputs_Previous = Control_Inputs_Initial; % The usual 'B' matrix but unused here.
Process_Model_Covariance_Matrix_Previous = Process_Model_Covariance_Matrix; % The 'Q' process model matrix.
Measurement_Covariance_Matrix_Previous = Measurement_Covariance_Matrix; % The 'R' measurement matrix.
Measurment_Current = [Position_Ship_X_Current_GPS,...
                      Position_Ship_Y_Current_GPS,...
                      Heading_GPS,...
                      Position_Ship_X_Current_INS,...
                      Position_Ship_Y_Current_INS,...
                      Heading_Current_INS,...
                      Heading_Magnetometer,...
                      Velocity_Ship_GPS,...
                      Velocity_Ship_INS];

% EKF loop calculation:
[State_Aposteriori_Current,Covariance_Aposteriori_Current] = EKF_Heading(States_Previous,Covariance_State_Previous,Control_Inputs_Previous,...
                                                                         Jacobian_State_Process_Model(States_Previous(4),States_Previous(3),Time_Step_Integration),...
                                                                         Process_Model_Covariance_Matrix_Previous,Measurement_Model_Matrix,...
                                                                         Measurement_Covariance_Matrix_Previous,...
                                                                         Function_Process_Model(States_Previous(1),States_Previous(2),States_Previous(3),States_Previous(4),Time_Step_Integration),...
                                                                         Measurment_Current');

% Inputs update:
State_Model_Prediction = State_Aposteriori_Current; % This must be stored and reused at the next step time.
Covariance_Model_Prediction = Covariance_Aposteriori_Current;

% Store the interesting components of the covariance matrix (diagonal
% terms):
Covariance_Position_X = Covariance_Aposteriori_Current(1,1);
Covariance_Position_Y = Covariance_Aposteriori_Current(2,2);
Covariance_Psi_Heading = Covariance_Aposteriori_Current(3,3);
Covariance_Velocity = Covariance_Aposteriori_Current(4,4);
Covariance_Error_Vector_Current = [Covariance_Position_X;...
                                   Covariance_Position_Y;...
                                   Covariance_Psi_Heading;...
                                   Covariance_Velocity];

% Filtered and fused data:
Position_Ship_X_Current_Filtered = State_Aposteriori_Current(1);
Position_Ship_Y_Current_Filtered = State_Aposteriori_Current(2);
Heading_Ship_Current_Filtered = State_Aposteriori_Current(3);
Velocity_Current_Filtered = State_Aposteriori_Current(4);

end

== matlab function Simulator_Case_7/Navigation_And_Wave_Estimator/Sensors_Fusion_And_Filtering/Real_Navigation_Sensors_Extended_Kalman_Filter/GPS_Sensor/LLA_To_ENU ==
  data: LLA_Coordinates input; ENU_GPS_Perturbed_Coordinates output
function ENU_GPS_Perturbed_Coordinates = Conversion_LLA_To_ENU(LLA_Coordinates)

% Reference point:
Reference_Point_Port_Mahon = [43.059023,3.002915,0];
Semi_Major_Axis = 6378137.0;
Flattening = 1/298.25;

% This function serves as a mean to convert LLA coordinates to ENU
% coordinates:
ENU_GPS_Perturbed_Coordinates = LLA_To_ENU(LLA_Coordinates(1),LLA_Coordinates(2),LLA_Coordinates(3),...
                                           Reference_Point_Port_Mahon(1),Reference_Point_Port_Mahon(2),...
                                           Reference_Point_Port_Mahon(3),Semi_Major_Axis,Flattening);


end

== matlab function Simulator_Case_7/Navigation_And_Wave_Estimator/Sensors_Fusion_And_Filtering/Real_Navigation_Sensors_Extended_Kalman_Filter/GPS_Sensor/Velocity_Norm_Calculation ==
  data: Velocity_Input_Vector_Current input; Velocity_Norm_Current output
function Velocity_Norm_Current = Velocity_Norm(Velocity_Input_Vector_Current)

Velocity_Norm_Current = sqrt(Velocity_Input_Vector_Current(1)^2 + Velocity_Input_Vector_Current(2)^2 + Velocity_Input_Vector_Current(3)^2);

end

== matlab function Simulator_Case_7/Environmental_Perturbations/Wind_Perturbation_Torque/Wind_Estimator ==
  data: Wind_Angle_Generated output; Wind_Velocity_Generated output; Wind_Speed output; Velocity_Ship input; Wind_Direction output; Table_Wind_Coefficients input; Yaw_Wind_Coefficient_Current output; Lenght_Ship_Overall input; Density_Air input; Area_Lateral_Projected_Wind input; Inertia_Ship_Vertical_Axis input; Heading_Induced_Wind output; Torque_Wind output; Time_Sampling input
function [Wind_Angle_Generated,...
          Wind_Velocity_Generated,...
          Wind_Speed,...
          Wind_Direction,...
          Yaw_Wind_Coefficient_Current,...
          Heading_Induced_Wind,...
          Torque_Wind] = Wind_Estimator(Velocity_Ship,...
                                        Table_Wind_Coefficients,...
                                        Lenght_Ship_Overall,...
                                        Density_Air,...
                                        Area_Lateral_Projected_Wind,...
                                        Inertia_Ship_Vertical_Axis,...
                                        Time_Sampling)

% Wind estimator and generator online algorithm:
[Wind_Angle_Generated,...
 Wind_Velocity_Generated,...
 Wind_Speed,...
 Wind_Direction,...
 Yaw_Wind_Coefficient_Current,...
 Heading_Induced_Wind,...
 Torque_Wind] = Wind_Estimator_Generator(Velocity_Ship,...
                                         Table_Wind_Coefficients,...
                                         Lenght_Ship_Overall,...
                                         Density_Air,...
                                         Area_Lateral_Projected_Wind,...
                                         Inertia_Ship_Vertical_Axis,...
                                         Time_Sampling);

end

== matlab function Simulator_Case_7/Navigation_And_Wave_Estimator/Wave_Identification_Parameters_ARMA ==
  data: Heading_Wave_High_Frequency_Estimated input; Wave_Pulsation_Estimated output; Wave_Damping_Factor_Estimated output; Time_Sampling input
function [Wave_Pulsation_Estimated,...
          Wave_Damping_Factor_Estimated] = Wave_Parameters_Identification_ARMA(Heading_Wave_High_Frequency_Estimated,...
                                                                               Time_Sampling)

% Two stage Recursive Extended least squares algorithm to estimate the wave
% pulsation and damping factor:
[Wave_Pulsation_Estimated,...
 Wave_Damping_Factor_Estimated] = Wave_Identification_ARMA(Heading_Wave_High_Frequency_Estimated,...
                                                           Time_Sampling);


end

== matlab function Simulator_Case_7/Navigation_And_Wave_Estimator/High_Pass_Filter ==
  data: Heading_Unfiltered_Input input; Heading_Filtered_Ouput output; Time_Sampling input
function Heading_Filtered_Ouput= High_Pass_Wave_Filter(Heading_Unfiltered_Input,...
                                                       Time_Sampling)

% Online numerical high-pass filter for pre-processing of the heading for
% identification:
Heading_Filtered_Ouput = High_Pass_Wave_Filter_Identification(Heading_Unfiltered_Input,...
                                                              Time_Sampling);

end

== matlab function Simulator_Case_7/Ship_Dynamics/Heading_Normalization_Function ==
  data: Heading_Input input; Heading_Normalized output
function Heading_Normalized = Heading_Normalization(Heading_Input)

% This function has the purpose of normalizing the heading angle avoiding
% non-physical values:
Heading_Normalized = mod(Heading_Input, 2*pi);

end

== matlab function Simulator_Case_7/Navigation_And_Wave_Estimator/Sensors_Fusion_And_Filtering/Real_Navigation_Sensors_Extended_Kalman_Filter/INS_Sensor/Velocity_Norm_Calculation ==
  data: Velocity_Input_Vector_Current input; Velocity_Norm_Current output
function Velocity_Norm_Current = Velocity_Norm(Velocity_Input_Vector_Current)

Velocity_Norm_Current = sqrt(Velocity_Input_Vector_Current(1)^2 + Velocity_Input_Vector_Current(2)^2 + Velocity_Input_Vector_Current(3)^2);

end

== matlab function Simulator_Case_7/Controller_And_Actuator/Ship_High_Level_Loop_Controller ==
  data: Heading_Aimed_Current input; Rudder_Angle_Elaborated_Current output; Heading_Observed_Current input; Gain_Proportional input; Gain_Filter input; Gain_Derivative input; Time_Sampling input
function Rudder_Angle_Elaborated_Current = PDF_Controller(Heading_Aimed_Current,...
                                                          Heading_Observed_Current,...
                                                          Gain_Proportional,...
                                                          Gain_Filter,...
                                                          Gain_Derivative,...
                                                          Time_Sampling)

% This is the Control algorithm written in the form of a simple discretized
% Proportional Derivative Filter (PDF). The discretization method used is
% the Tustin Bilinear Transform.
Rudder_Angle_Elaborated_Current = Controller_PDF_Algorithm(Heading_Aimed_Current,...
                                                           Heading_Observed_Current,...
                                                           Gain_Proportional,...
                                                           Gain_Filter,...
                                                           Gain_Derivative,...
                                                           Time_Sampling);

end

== matlab function Simulator_Case_7/Guidance_Heading/Guidance_Algorithm ==
  settings: updateMethod=DISCRETE
  data: Velocity_Current input; Heading_Aimed_Next output; Waypoints input; Position_X_Ship_Current input; Position_Y_Ship_Current input; Heading_Ship_Current input; Position_X_Final_Waypoint input; Position_Y_Final_Waypoint input; Time_Current input; Time_End_Guidance output
function [Heading_Aimed_Next,Time_End_Guidance] = Guidance_Waypoints_Following(Velocity_Current,...
                                                                               Waypoints,...
                                                                               Position_X_Ship_Current,...
                                                                               Position_Y_Ship_Current,...
                                                                               Heading_Ship_Current,...
                                                                               Position_X_Final_Waypoint,...
                                                                               Position_Y_Final_Waypoint,...
                                                                               Time_Current)

% Call of the final embedded Guidance function based on Waypoints
% following:
[Heading_Aimed_Next,Time_End_Guidance] = Guidance_Waypoints_Following_Embedded(Velocity_Current,...
                                                                               Waypoints,...
                                                                               Position_X_Ship_Current,...
                                                                               Position_Y_Ship_Current,...
                                                                               Heading_Ship_Current,...
                                                                               Position_X_Final_Waypoint,...
                                                                               Position_Y_Final_Waypoint,...
                                                                               Time_Current);
end

== matlab function Simulator_Case_7/Controller_And_Actuator/Actuator_Control ==
  data: Rudder_Commanded_High_Level_Loop_Current input; Rudder_Commanded_Elaborated_Current output; Rudder_Angle_Maximal input; Rudder_Angle_Minimal input; Rudder_Rate_Maximal input; Rudder_Rate_Minimal input; Time_Sampling input
function Rudder_Commanded_Elaborated_Current = Linear_Actuator_First_Order(Rudder_Commanded_High_Level_Loop_Current,...
                                                                           Rudder_Angle_Maximal,...
                                                                           Rudder_Angle_Minimal,...
                                                                           Rudder_Rate_Maximal,...
                                                                           Rudder_Rate_Minimal,...
                                                                           Time_Sampling)

% This function acts as a simplified model of a first Actuator version. It
% consists in a first saturation of the commanded rudder angle in terms of
% maximal and minimal angles value. And a second saturation in terms of maximal and
% minimal rudder angle rate.
Rudder_Commanded_Elaborated_Current = Rudder_Angle_Rate_Saturations(Rudder_Commanded_High_Level_Loop_Current,...
                                                                    Rudder_Angle_Maximal,...
                                                                    Rudder_Angle_Minimal,...
                                                                    Rudder_Rate_Maximal,...
                                                                    Rudder_Rate_Minimal,...
                                                                    Time_Sampling);

end
